simulink subsystem "Distance_LED_Bhv"  (R2023b)
settings: Solver=VariableStepAuto  StartTime=0.0  StopTime=10.0  RelTol=1e-3
settings Model: Creator=m4ttn  LastModifiedBy=m4ttn

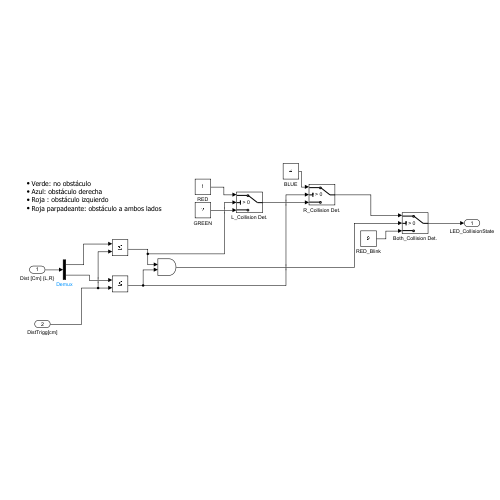
[thumbnail: Simulink's stored preview of the top-level diagram]
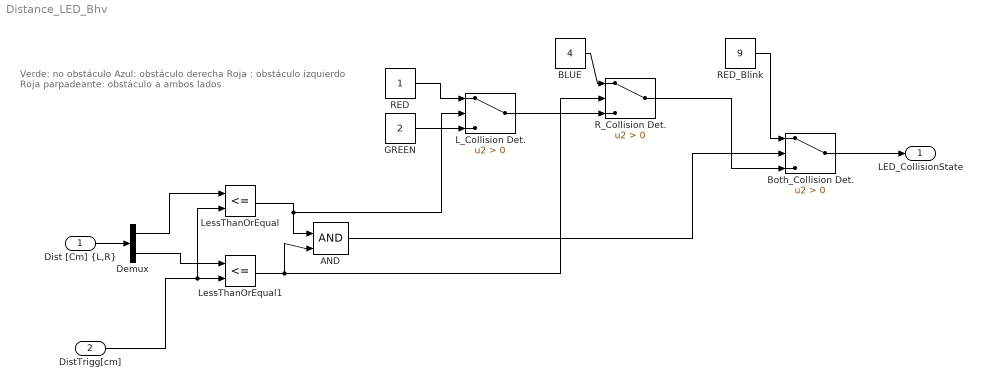
== system Distance_LED_Bhv ==
  note: Verde: no obstáculo
      | Azul: obstáculo derecha
      | Roja : obstáculo izquierdo
      | Roja parpadeante: obstáculo a ambos lados
  "Dist [Cm] {L,R}" : Inport  OutDataTypeStr=uint8
  DistTrigg[cm] : Inport  Port=2
  AND : Logic  IconShape=distinctive  AllPortsSameDT=off  OutDataTypeStr=boolean
  BLUE : Constant  Value=4  OutDataTypeStr=uint8
  Both_Collision Det. : Switch  Criteria=u2 > Threshold  OutDataTypeStr=uint8  SaturateOnIntegerOverflow=off  InputSameDT=off
  Demux : Demux  Outputs=2
  GREEN : Constant  Value=2  OutDataTypeStr=uint8
  L_Collision Det. : Switch  Criteria=u2 > Threshold  OutDataTypeStr=uint8  SaturateOnIntegerOverflow=off  InputSameDT=off
  LessThanOrEqual : RelationalOperator  Operator=<=  OutDataTypeStr=boolean  RndMeth=Simplest  InputSameDT=off
  LessThanOrEqual1 : RelationalOperator  Operator=<=  OutDataTypeStr=boolean  RndMeth=Simplest  InputSameDT=off
  RED : Constant  OutDataTypeStr=uint8
  RED_Blink : Constant  Value=9  OutDataTypeStr=uint8
  R_Collision Det. : Switch  Criteria=u2 > Threshold  OutDataTypeStr=uint8  SaturateOnIntegerOverflow=off  InputSameDT=off
  LED_CollisionState : Outport  OutDataTypeStr=uint8
  wires:
  "Dist [Cm] {L,R}"/1 -> Demux/1
  Demux/1 -> LessThanOrEqual/1
  Demux/2 -> LessThanOrEqual1/1
  DistTrigg[cm]/1 -> LessThanOrEqual/2, LessThanOrEqual1/2
  LessThanOrEqual/1 -> L_Collision Det./2, AND/1
  LessThanOrEqual1/1 -> R_Collision Det./2, AND/2
  GREEN/1 -> L_Collision Det./3
  R_Collision Det./1 -> Both_Collision Det./3
  L_Collision Det./1 -> R_Collision Det./3
  AND/1 -> Both_Collision Det./2
  RED_Blink/1 -> Both_Collision Det./1
  RED/1 -> L_Collision Det./1
  BLUE/1 -> R_Collision Det./1
  Both_Collision Det./1 -> LED_CollisionState/1
